simulink model "mars_rover_ex_1b"  (R2023a)
settings: Solver=ode23t  StartTime=0.0  StopTime=Rover.simStopTimeEx1b  FixedStep=1e-2  MaxStep=0.1  RelTol=1e-3  AbsTol=1e-3  EnableMultiTasking=on
StartFcn:
  | mars_rover_ex1b_sim_callback
model workspace (MATLAB code in the model file):
  | addpath("mars_rover_helpers");
  | % Load Rover Arm model for IK
  | mdlpath = ['mars_rover_data',filesep,'mars_rover_arm'];
  | load_system(mdlpath);
  | 
  | imdata = zeros(3,3,3);
  | 
  | % Temp
  | Kp_steer = 1;
  | Ki_steer = 1;
  | Kd_steer = 1;
  | 
  | Kp = 1;
  | Ki = 1;
  | Kd = 1;
values from neighbouring files (symbols this model uses):
  cam_base_angle = 0    [mars_rover_params.m]
  cam_target_angle = 20    [mars_rover_params.m]
  mapData = false(197,200)    [mars_rover_params.m]    (also in mars_rover_startup.m)
  roverPath = app.rover_path    [NavigateOnMars.m]    (also in mars_rover_params.m = rover_path1)
undefined symbols (not defined in the file or in its folder): Arm, armJointAng, armJointTrqs, cameraData, eeConfig, pose, Rover, rover_path_ex1, sampleLocation, steerAng, steerTrqs, Terrain, vSpeed, Wheel1_G, Wheel2_G, Wheel3_G, Wheel4_G, Wheel5_G, Wheel6_G, wheelTrqs, wSpeeds, X, Y, Z
libraries: sm_lib x238, nesl_utility x80, slpidlib x3, simulink x3, simulink_extras x2, robotcorelib x1, robotalgslib x1
(part 9 of 9)

== system mars_rover_ex_1b/Mars Rover Plant/Rover Plant Model/Rover /Wheels/SteeringBracketLF ==
  File Solid5 : sm_lib/Body Elements/File Solid  ExtGeomFileName=mobility_steering_bracket.stl  UnitType=Custom  ExtGeomFileUnits=cm  StepReaderType=HEX  ExportConvexHullGeometry=off  InertiaType=CalculateFromGeometry  Mass=0  MassUnits=kg  CenterOfMass=[0 0 0]  CenterOfMassUnits=m  MomentsOfInertia=[1 1 1]*0  MomentsOfInertiaUnits=kg*m^2  ProductsOfInertia=[0 0 0]  ProductsOfInertiaUnits=kg*m^2  BasedOnType=Density  Density=1000  DensityUnits=kg/m^3  DoExposeReferenceFrame=on  SerializedFrames=<Frames/>  GraphicType=FromGeometry  MarkerShape=Sphere  MarkerSize=10  GraphicVisPropType=AdvancedVisualProperties  GraphicDiffuseColor=[0.2 0.2 0.2]  GraphicSpecularColor=[1 1 1 1.0]  GraphicAmbientColor=[0.15 0.15 0.15 1.0]  GraphicEmissiveColor=[0.0 0.0 0.0 1.0]  GraphicShininess=90  GraphicOpacity=1.0
  Reference Frame : sm_lib/Frames and Transforms/Reference Frame
  Rigid Transform : sm_lib/Frames and Transforms/Rigid Transform  TranslationMethod=Cartesian  TranslationStandardOffset=0  TranslationStandardOffsetUnits=m  TranslationStandardAxis=+Z  TranslationCartesianOffset=Rover.SB.SRJ_T  TranslationCartesianOffsetUnits=m  TranslationROffset=0  TranslationROffsetUnits=m  TranslationZOffset=0  TranslationZOffsetUnits=m  TranslationThetaOffset=0  TranslationThetaOffsetUnits=deg  RotationMethod=RotationMatrix  RotationAngleUnits=deg  RotationStandardAxis=+Z  RotationAngle=0.0  RotationArbitraryAxis=[0 0 1]  FollAlignAxisA=+X  BaseAlignAxisA=+Y  FollAlignAxisB=+Y  BaseAlignAxisB=+Z  RotationSequenceAxes=FollowerAxes  RotationSequence=XYX  RotationSequenceAngles=[0 0 0]  RotationSequenceAnglesUnits=deg  RotationMatrix=Rover.SB.SRJ_R  Quaternion=[1 0 0 0]
  Rigid Transform1 : sm_lib/Frames and Transforms/Rigid Transform  TranslationMethod=Cartesian  TranslationStandardOffset=0  TranslationStandardOffsetUnits=m  TranslationStandardAxis=+Z  TranslationCartesianOffset=Rover.SB.WRJ_T  TranslationCartesianOffsetUnits=m  TranslationROffset=0  TranslationROffsetUnits=m  TranslationZOffset=0  TranslationZOffsetUnits=m  TranslationThetaOffset=0  TranslationThetaOffsetUnits=deg  RotationMethod=RotationMatrix  RotationAngleUnits=deg  RotationStandardAxis=+Z  RotationAngle=0.0  RotationArbitraryAxis=[0 0 1]  FollAlignAxisA=+X  BaseAlignAxisA=+Y  FollAlignAxisB=+Y  BaseAlignAxisB=+Z  RotationSequenceAxes=FollowerAxes  RotationSequence=XYX  RotationSequenceAngles=[0 0 0]  RotationSequenceAnglesUnits=deg  RotationMatrix=Rover.SB.WRJ_R  Quaternion=[1 0 0 0]
  SRJ : PMIOPort  Side=Left
  WRJ : PMIOPort  Port=2  Side=Right
  connections:
  Rigid Transform/RConn1 -- SRJ/RConn1
  WRJ/RConn1 -- Rigid Transform1/RConn1
  File Solid5/RConn1 -- Reference Frame/RConn1 -- Rigid Transform1/LConn1 -- Rigid Transform/LConn1

== system mars_rover_ex_1b/Mars Rover Plant/Rover Plant Model/Rover /Wheels/SteeringBracketRB ==
  File Solid5 : sm_lib/Body Elements/File Solid  ExtGeomFileName=mobility_steering_bracket.stl  UnitType=Custom  ExtGeomFileUnits=cm  StepReaderType=HEX  ExportConvexHullGeometry=off  InertiaType=CalculateFromGeometry  Mass=0  MassUnits=kg  CenterOfMass=[0 0 0]  CenterOfMassUnits=m  MomentsOfInertia=[1 1 1]*0  MomentsOfInertiaUnits=kg*m^2  ProductsOfInertia=[0 0 0]  ProductsOfInertiaUnits=kg*m^2  BasedOnType=Density  Density=1000  DensityUnits=kg/m^3  DoExposeReferenceFrame=on  SerializedFrames=<Frames/>  GraphicType=FromGeometry  MarkerShape=Sphere  MarkerSize=10  GraphicVisPropType=AdvancedVisualProperties  GraphicDiffuseColor=[0.2 0.2 0.2]  GraphicSpecularColor=[1 1 1 1.0]  GraphicAmbientColor=[0.15 0.15 0.15 1.0]  GraphicEmissiveColor=[0.0 0.0 0.0 1.0]  GraphicShininess=90  GraphicOpacity=1.0
  Reference Frame : sm_lib/Frames and Transforms/Reference Frame
  Rigid Transform : sm_lib/Frames and Transforms/Rigid Transform  TranslationMethod=Cartesian  TranslationStandardOffset=0  TranslationStandardOffsetUnits=m  TranslationStandardAxis=+Z  TranslationCartesianOffset=Rover.SB.SRJ_T  TranslationCartesianOffsetUnits=m  TranslationROffset=0  TranslationROffsetUnits=m  TranslationZOffset=0  TranslationZOffsetUnits=m  TranslationThetaOffset=0  TranslationThetaOffsetUnits=deg  RotationMethod=RotationMatrix  RotationAngleUnits=deg  RotationStandardAxis=+Z  RotationAngle=0.0  RotationArbitraryAxis=[0 0 1]  FollAlignAxisA=+X  BaseAlignAxisA=+Y  FollAlignAxisB=+Y  BaseAlignAxisB=+Z  RotationSequenceAxes=FollowerAxes  RotationSequence=XYX  RotationSequenceAngles=[0 0 0]  RotationSequenceAnglesUnits=deg  RotationMatrix=Rover.SB.SRJ_R  Quaternion=[1 0 0 0]
  Rigid Transform1 : sm_lib/Frames and Transforms/Rigid Transform  TranslationMethod=Cartesian  TranslationStandardOffset=0  TranslationStandardOffsetUnits=m  TranslationStandardAxis=+Z  TranslationCartesianOffset=Rover.SB.WRJ_T  TranslationCartesianOffsetUnits=m  TranslationROffset=0  TranslationROffsetUnits=m  TranslationZOffset=0  TranslationZOffsetUnits=m  TranslationThetaOffset=0  TranslationThetaOffsetUnits=deg  RotationMethod=RotationMatrix  RotationAngleUnits=deg  RotationStandardAxis=+Z  RotationAngle=0.0  RotationArbitraryAxis=[0 0 1]  FollAlignAxisA=+X  BaseAlignAxisA=+Y  FollAlignAxisB=+Y  BaseAlignAxisB=+Z  RotationSequenceAxes=FollowerAxes  RotationSequence=XYX  RotationSequenceAngles=[0 0 0]  RotationSequenceAnglesUnits=deg  RotationMatrix=Rover.SB.WRJ_R  Quaternion=[1 0 0 0]
  SRJ : PMIOPort  Side=Left
  WRJ : PMIOPort  Port=2  Side=Right
  connections:
  Rigid Transform/LConn1 -- Rigid Transform1/LConn1 -- Reference Frame/RConn1 -- File Solid5/RConn1
  WRJ/RConn1 -- Rigid Transform1/RConn1
  Rigid Transform/RConn1 -- SRJ/RConn1

== system mars_rover_ex_1b/Mars Rover Plant/Rover Plant Model/Rover /Wheels/SteeringBracketRF ==
  File Solid5 : sm_lib/Body Elements/File Solid  ExtGeomFileName=mobility_steering_bracket.stl  UnitType=Custom  ExtGeomFileUnits=cm  StepReaderType=HEX  ExportConvexHullGeometry=off  InertiaType=CalculateFromGeometry  Mass=0  MassUnits=kg  CenterOfMass=[0 0 0]  CenterOfMassUnits=m  MomentsOfInertia=[1 1 1]*0  MomentsOfInertiaUnits=kg*m^2  ProductsOfInertia=[0 0 0]  ProductsOfInertiaUnits=kg*m^2  BasedOnType=Density  Density=1000  DensityUnits=kg/m^3  DoExposeReferenceFrame=on  SerializedFrames=<Frames/>  GraphicType=FromGeometry  MarkerShape=Sphere  MarkerSize=10  GraphicVisPropType=AdvancedVisualProperties  GraphicDiffuseColor=[0.2 0.2 0.2]  GraphicSpecularColor=[1 1 1 1.0]  GraphicAmbientColor=[0.15 0.15 0.15 1.0]  GraphicEmissiveColor=[0.0 0.0 0.0 1.0]  GraphicShininess=90  GraphicOpacity=1.0
  Reference Frame : sm_lib/Frames and Transforms/Reference Frame
  Rigid Transform : sm_lib/Frames and Transforms/Rigid Transform  TranslationMethod=Cartesian  TranslationStandardOffset=0  TranslationStandardOffsetUnits=m  TranslationStandardAxis=+Z  TranslationCartesianOffset=Rover.SB.SRJ_T  TranslationCartesianOffsetUnits=m  TranslationROffset=0  TranslationROffsetUnits=m  TranslationZOffset=0  TranslationZOffsetUnits=m  TranslationThetaOffset=0  TranslationThetaOffsetUnits=deg  RotationMethod=RotationMatrix  RotationAngleUnits=deg  RotationStandardAxis=+Z  RotationAngle=0.0  RotationArbitraryAxis=[0 0 1]  FollAlignAxisA=+X  BaseAlignAxisA=+Y  FollAlignAxisB=+Y  BaseAlignAxisB=+Z  RotationSequenceAxes=FollowerAxes  RotationSequence=XYX  RotationSequenceAngles=[0 0 0]  RotationSequenceAnglesUnits=deg  RotationMatrix=Rover.SB.SRJ_R  Quaternion=[1 0 0 0]
  Rigid Transform1 : sm_lib/Frames and Transforms/Rigid Transform  TranslationMethod=Cartesian  TranslationStandardOffset=0  TranslationStandardOffsetUnits=m  TranslationStandardAxis=+Z  TranslationCartesianOffset=Rover.SB.WRJ_T  TranslationCartesianOffsetUnits=m  TranslationROffset=0  TranslationROffsetUnits=m  TranslationZOffset=0  TranslationZOffsetUnits=m  TranslationThetaOffset=0  TranslationThetaOffsetUnits=deg  RotationMethod=RotationMatrix  RotationAngleUnits=deg  RotationStandardAxis=+Z  RotationAngle=0.0  RotationArbitraryAxis=[0 0 1]  FollAlignAxisA=+X  BaseAlignAxisA=+Y  FollAlignAxisB=+Y  BaseAlignAxisB=+Z  RotationSequenceAxes=FollowerAxes  RotationSequence=XYX  RotationSequenceAngles=[0 0 0]  RotationSequenceAnglesUnits=deg  RotationMatrix=Rover.SB.WRJ_R  Quaternion=[1 0 0 0]
  SRJ : PMIOPort  Side=Left
  WRJ : PMIOPort  Port=2  Side=Right
  connections:
  Rigid Transform/RConn1 -- SRJ/RConn1
  WRJ/RConn1 -- Rigid Transform1/RConn1
  File Solid5/RConn1 -- Reference Frame/RConn1 -- Rigid Transform1/LConn1 -- Rigid Transform/LConn1

== system mars_rover_ex_1b/Mars Rover Plant/Rover Plant Model/Rover Pose Sensing/Kalman Filter/accelerometer ==
  Constant3 : Constant  Value=[0 0 3.72076]
  Ideal Sensor : sm_lib/Frames and Transforms/Transform Sensor  MeasurementFrame=NonRotatingFollower  RotationSequence=XYX  SenseAngle=off  SenseAxis=off  SenseQ=off  SenseR=on  SenseRotationSequence=off  SenseOmegaX=off  SenseOmegaY=off  SenseOmegaZ=off  SenseQDot=off  SenseRDot=off  SenseRotationSequenceDot=off  SenseAlphaX=off  SenseAlphaY=off  SenseAlphaZ=off  SenseQDDot=off  SenseRDDot=off  SenseX=off  SenseY=off  SenseZ=off  SenseRad=off  SenseAzim=off  SenseDist=off  SenseInc=off  SenseXDot=off  SenseYDot=off  SenseZDot=off  SenseRadDot=off  SenseAzimDot=off  SenseDistDot=off  SenseIncDot=off  SenseXDDot=on  SenseYDDot=on  SenseZDDot=on  SenseRadDDot=off  SenseAzimDDot=off  SenseDistDDot=off  SenseIncDDot=off
  Matrix Multiply : Product  Multiplication=Matrix(*)
  Mux : Mux  Inputs=3
  PS-Simulink Converter{6,8..10} (4 alike) : nesl_utility/PS-Simulink Converter  PhysicalDomain=network_engine_domain  SubClassName=ps_output  LeftPortType=input  RightPortType=output  PseudoPeriodic=off  Frequencies=[]  VectorFormat=inherit  Unit=inherit  AffineConversion=off
  Sensor Noise : RandomNumber  Variance=0.01  SampleTime=1
  Sum : Sum  Inputs=++|
  Sum1 : Sum  Inputs=++|
  Transpose : Math  Operator=transpose
  Rover : PMIOPort  Side=Right
  World : PMIOPort  Port=2  Side=Left
  Accelerometer Readings : Outport
  Direction Cosine Matrix : Outport  Port=2
  wires:
  PS-Simulink Converter9/1 -> Mux/3
  Mux/1 -> Sum/2
  Matrix Multiply/1 -> Sum/1
  PS-Simulink Converter6/1 -> Mux/1
  PS-Simulink Converter10/1 -> Direction Cosine Matrix/1, Transpose/1
  PS-Simulink Converter8/1 -> Mux/2
  Transpose/1 -> Matrix Multiply/1
  Constant3/1 -> Matrix Multiply/2
  Sensor Noise/1 -> Sum1/1
  Sum/1 -> Sum1/2
  Sum1/1 -> Accelerometer Readings/1
  connections:
  PS-Simulink Converter10/LConn1 -- Ideal Sensor/RConn2
  PS-Simulink Converter8/LConn1 -- Ideal Sensor/RConn4
  PS-Simulink Converter9/LConn1 -- Ideal Sensor/RConn5
  Ideal Sensor/RConn1 -- Rover/RConn1
  PS-Simulink Converter6/LConn1 -- Ideal Sensor/RConn3
  Ideal Sensor/LConn1 -- World/RConn1

== system mars_rover_ex_1b/Control/Rover Control/Rover Path Planning And Control/hold/RoverStopTime/Enabled Subsystem1 ==
  In1 : Inport
  Enable : EnablePort
  Out1 : Outport
  wires:
  In1/1 -> Out1/1

== matlab function mars_rover_ex_1b/Mars Rover Plant/Rover Plant Model/Rover Pose Sensing/Kalman Filter/Pose Estimation Outputs ==
  settings: updateMethod=DISCRETE  sampleTime=10
  data: plannedPath input; plannedPath_out output; estimatedXYStates input; estimatedXYStates_out output
function [plannedPath_out, estimatedXYStates_out]= fcn(plannedPath,estimatedXYStates)

plannedPath_out = plannedPath;
estimatedXYStates_out = estimatedXYStates;
end

== matlab function mars_rover_ex_1b/Control/Rover Control/Rover Path Planning And Control/Trapezoidal Vel Profile ==
  data: linVel input; t input; t1 input; lin_Vel_out output; accel input; deaccelStartTime input
function lin_Vel_out = fcn(linVel,t,t1,accel,deaccelStartTime)
% Function to create a trapezoidal profile for rover's desired linear
% velocity

t2 = linVel/accel + t1;
t3 = deaccelStartTime + 0.2;
tf = linVel/accel + t3;

if t>=t1 && t<t2 
    lin_Vel_out = accel*(t-t1);

elseif t>=t2 && t < t3 
    lin_Vel_out = linVel;

elseif t>= t3 && t < tf 
    lin_Vel_out = linVel-accel*(t-t3);

else
    lin_Vel_out = 0;    
end


end

== matlab function mars_rover_ex_1b/Control/Rover Control/Rover Path Planning And Control/Ackerman Steer Angle/Ackerman Steering Angle Formulation ==
  data: delta input; LFsteerAng output; L input; RFsteerAng output; d input; R output; L_R output; R_R output
function [LFsteerAng,RFsteerAng,R,L_R,R_R] = fcn(delta,L,d)
% Function to compute ackerman steering angles from a bicycle steer angle.

R = L/tand(abs(delta));

if delta < 0
    LFsteerAng = atan2d(L,(R+d/2));
    RFsteerAng = atan2d(L,(R-d/2));
    L_R = (R+d/2);
    R_R = (R-d/2);
else
    LFsteerAng = -atan2d(L,(R-d/2));
    RFsteerAng = -atan2d(L,(R+d/2));
    L_R = (R-d/2);
    R_R = (R+d/2);
end

end

== matlab function mars_rover_ex_1b/Control/Rover Control/Rover Path Planning And Control/Chassis Velocity To Wheel Speed ==
  data: desChassisSpeed input; wheel_speed_LF output; wheel_r input; steer_ang input; wheel_speed_LM output; wheel_speed_LB output; R input; L input; L_R input; R_R input; wheel_speed_RF output; wheel_speed_RM output; wheel_speed_RB output
function [wheel_speed_LF,wheel_speed_LM,wheel_speed_LB,...
    wheel_speed_RF,wheel_speed_RM,wheel_speed_RB] = fcn(desChassisSpeed,wheel_r,steer_ang,R,L,L_R,R_R)
% Function to compute wheel speed from a desired linear velocity and
% desired path.

if any(abs(steer_ang) > 0)

    wheel_speed_LF = (desChassisSpeed/wheel_r)*sqrt(L_R^2 + L^2)/R;
    wheel_speed_LM = desChassisSpeed * L_R/(R*wheel_r);
    wheel_speed_LB = (desChassisSpeed/wheel_r)*sqrt(L_R^2 + L^2)/R;
    wheel_speed_RF = -(desChassisSpeed/wheel_r)*sqrt(R_R^2 + L^2)/R;
    wheel_speed_RM = -desChassisSpeed * R_R/(R*wheel_r);
    wheel_speed_RB = -(desChassisSpeed/wheel_r)*sqrt(R_R^2 + L^2)/R;

else
    wheel_speed_LF = desChassisSpeed / wheel_r;
    wheel_speed_LM = desChassisSpeed / wheel_r;
    wheel_speed_LB = desChassisSpeed / wheel_r;
    wheel_speed_RF = -desChassisSpeed / wheel_r;
    wheel_speed_RM = -desChassisSpeed / wheel_r;
    wheel_speed_RB = -desChassisSpeed / wheel_r;
end

end

== matlab function mars_rover_ex_1b/Control/Manipulator Control/ Trajectory Planner/Planner Subsystem/Task Scheduler ==
  settings: updateMethod=DISCRETE
  data: wayPts output; reset_t output; samplePickCmd output; sampleDropCmd output; actJointAngles input; desJointAngles input; samplePickSense input; sampleDropSense input; currentTime input; stop output
function [wayPts,reset_t,samplePickCmd,sampleDropCmd,stop]  = fcn(actJointAngles,desJointAngles,samplePickSense,sampleDropSense,currentTime)
% This function plans the top level tasks for the arm. The end effector goal
% and sample interaction joint configuration modes depend on the current task mode.
%
% mode 0: home/initial position (waypt 1) (samplePickCmd Off)
% mode 1-2: move to the position close the sample (waypt 3 via waypt 2) (samplePickCmd Off)
% mode 3-4 : move to sample position and pick up sample (waypt 4) (samplePickCmd On)
% mode 5 : move back to the position close the sample (waypt 3) (samplePickCmd On)
% mode 6 : move to the position close to the sample storage unit (waypt 5) (samplePickCmd On)
% mode 7-8 : move to sample storage position and drop/collect sample (waypt 6) (sampleDropCmd On)
% mode 9 : move back to the position close to the sample storage unit (samplePickCmd,sampleDropCmd On)
% mode 10-11 :move to home position 

maxErrPos = 0.5;
actJointAngles =actJointAngles';
persistent mode resetTime
stop = 0;
if isempty(mode)
    mode = 0;
    resetTime = 0;
end

reset_t =  resetTime;

switch mode

    case 0
        % Home Position
        wayPts = [desJointAngles(1,:);desJointAngles(1,:)];
        samplePickCmd = false;
        sampleDropCmd = false;

        if all(abs(actJointAngles-desJointAngles(1,:)) < maxErrPos)
            resetTime = currentTime;
            if sampleDropSense == 1
                mode = 0;
            else
                mode = 1;
            end
        end

    case 1
        
        wayPts = desJointAngles(1:2,:);
        samplePickCmd = false;
        sampleDropCmd = false;

        if all(abs(actJointAngles-desJointAngles(2,:)) < maxErrPos)
            resetTime = currentTime;
            mode = 2;
        end

    case 2
        % Move to the position close the sample
        wayPts = desJointAngles(2:3,:);
        samplePickCmd = false;
        sampleDropCmd = false;

        if all(abs(actJointAngles-desJointAngles(3,:)) < maxErrPos)
            resetTime = currentTime;
            mode = 3;
        end

    case 3
        % Move to sample position
        wayPts = desJointAngles(3:4,:);
        samplePickCmd = false;
        sampleDropCmd = false;

        if all(abs(actJointAngles-desJointAngles(4,:)) < maxErrPos)
            resetTime = currentTime;
            mode = 4;
        end

    case 4
        % Stay at sample position and pick up the sample
        wayPts = [desJointAngles(4,:); desJointAngles(4,:)];
        samplePickCmd = true;
        sampleDropCmd = false;

        if all(abs(actJointAngles-desJointAngles(4,:)) < maxErrPos) && samplePickSense == 1
            resetTime = currentTime;
            mode = 5;
        end

    case 5
        % Move back to the position close to the sample
        wayPts = desJointAngles(4:-1:3,:);
        samplePickCmd = true;
        sampleDropCmd = false;

        if all(abs(actJointAngles-desJointAngles(3,:)) < maxErrPos)
            resetTime = currentTime;
            mode = 6;
        end


    case 6
        % Move the position close to the sample storage unit
        wayPts = [desJointAngles(3,:) ;desJointAngles(5,:)];
        samplePickCmd = true;
        sampleDropCmd = false;

        if all(abs(actJointAngles-desJointAngles(5,:)) < maxErrPos)
            resetTime = currentTime;
            mode = 7;
        end

    case 7
        % Move to the sample storage unit position
        wayPts = desJointAngles(5:6,:);
        sampleDropCmd = false;
        samplePickCmd = true;

        if all(abs(actJointAngles-desJointAngles(6,:)) < maxErrPos)
            resetTime = currentTime;
            mode = 8;
        end

    case 8
        % Stay at sample drop position, drop and collect the sample
        wayPts = [desJointAngles(6,:);desJointAngles(6,:)];

        sampleDropCmd = true;
        samplePickCmd = true;

        if (all(abs(actJointAngles-desJointAngles(6,:)) < maxErrPos)) && sampleDropSense == 1
            resetTime = currentTime;
            mode = 9;
        end

    case 9
        % Move back to the position close to the sample storage unit
        wayPts = desJointAngles(6:-1:5,:);
        sampleDropCmd = true;
        samplePickCmd = true;

        if all(abs(actJointAngles-desJointAngles(5,:)) < maxErrPos)
            resetTime = currentTime;
            mode = 10;
        end

    case 10
        % Move to home position via waypt 2
        wayPts = [desJointAngles(5,:); desJointAngles(7,:)];
        sampleDropCmd = true;
        samplePickCmd = true;

        if all(abs(actJointAngles-desJointAngles(7,:)) < maxErrPos)
            resetTime = currentTime;
            mode = 11;
        end

    case 11
        % Move to home position
        wayPts = [desJointAngles(7,:); desJointAngles(1,:)];
        sampleDropCmd = true;
        samplePickCmd = true;

        if all(abs(actJointAngles-desJointAngles(1,:)) < maxErrPos)
            resetTime = currentTime;           
            mode = 12;
        end
   
    case 12
        % Mission Complete
        wayPts = [desJointAngles(7,:); desJointAngles(1,:)];
        sampleDropCmd = true;
        samplePickCmd = true;
        mode = 12;
        stop = 1;
    otherwise
        error('invalid mode');

end

end

== matlab function mars_rover_ex_1b/Control/Manipulator Control/ Trajectory Planner/Planner Subsystem/Inverse Kinematics ==
  data: jointSpaceWayPts output; eePoseDes input; eeIgs input; samplePosition input; prevWayPts input
function  jointSpaceWayPts = fcn(eePoseDes,eeIgs,samplePosition,prevWayPts)
% Wrapper around sm_mars_rover_arm_ik.m
% Takes end effector targets and initial guesses and returns all the
% actuator positions corresponding to each target.

coder.extrinsic("mars_rover_arm_ik");

jointSpaceWayPts = zeros(7,6); %#ok<PREALL> 

% End effector Targets and initial guesses derived from sample location
samplePose = [samplePosition 175 0 91];
sample_position_eef = samplePose;
sample_position_eef_ig = [90.0000 -200.0000   90.0000   40.0000  170.0000  -10.0000];%[90   -200  160  90 170 -60];
sample_pos_init_eef = [sample_position_eef(1) sample_position_eef(2) sample_position_eef(3)+0.1 sample_position_eef(4) sample_position_eef(5) sample_position_eef(6)];
sample_pos_init_eef_ig = [90.0000 -200.0000   90.0000   40.0000  170.0000  -10.0000];%[90   -200  160  90 170 0];

% Combine precomputed end effector targets (waypts 1,2,5,6) with the
% ones derived from sample location (waypts 3,4) to create a set of
% task space waypoints for planning the trajectory.

EndEffTargets = ... 
    [eePoseDes(1,:);...% Waypt 1,(HomePos)
     eePoseDes(2,:);...% Waypt 2
    sample_pos_init_eef;...% Waypt 3,(Position near sample)
    sample_position_eef;...% Waypt 4 (Sample position)
    eePoseDes(3,:);... % Waypt 5,(Position near storage unit)
    eePoseDes(4,:);...% Waypt 6,(Sample storage position)
    eePoseDes(5,:);...
    ];

EndEffIgs = ...
     [eeIgs(1,:);...
     eeIgs(2,:);...
     sample_pos_init_eef_ig ;...  
     sample_position_eef_ig;...
     eeIgs(3,:);...
     eeIgs(4,:);...
     eeIgs(5,:);...
    ];

% Obtain joint space waypoints by calling IK for each end effector target
if prevWayPts == zeros(7,6)
[jointSpaceWayPts,solvedFlag] =  mars_rover_arm_ik(EndEffTargets,EndEffIgs); %#ok<ASGLU> 
else
jointSpaceWayPts = prevWayPts;
end

end

== matlab function mars_rover_ex_1b/Mars Rover Plant/Manipulator Plant Model/SampleGeneration/Subsystem/MATLAB Function ==
  data: roverPose input; sampleLoc output; terrainPts input
function sampleLoc = fcn(roverPose,terrainPts)
sampleLoc = zeros(3,1);
coder.extrinsic("scatteredInterpolant");

    P_rs = [2.25; 0; 0];
    R_wr = eul2rotm([0 0 roverPose(3)],'XYZ');
    P_wr = [roverPose(1) roverPose(2) 0];

    P_ws = P_wr' + R_wr*P_rs;

    F = scatteredInterpolant(terrainPts(:,1),terrainPts(:,2),terrainPts(:,3));
    sampleLoc = [P_ws(1);P_ws(2);F(P_ws(1),P_ws(2))];


end

== matlab function mars_rover_ex_1b/Mars Rover Plant/Rover Plant Model/Rover Pose Sensing/Kalman Filter/Discrete-Time Linear Kalman Filter ==
  settings: updateMethod=DISCRETE  sampleTime=1
  data: accelerometerData input; EstPose output; DCMMat input; rover_initialPosition input; t input; wheelSpeed input; wheel_radius input; EstLinVel output; EstLinAccel output; linVelocity input
function [EstPose, EstLinVel, EstLinAccel]  = fcn(accelerometerData, DCMMat,rover_initialPosition, t, wheelSpeed, wheel_radius,linVelocity)
% Discrete-Time Kalman Filter Block to estimate the position, linear
% velocity and linear acceleration of the rover using the IMU data and
% wheel speed. The system is defined as follows in continuous time: x_dot =
% [0 0 0 1 0 0 0 0 0; 0 0 0 0 1 0 0 0 0; 0 0 0 0 0 1 0 0 0;...
%          0 0 0 0 0 0 1 0 0; 0 0 0 0 0 0 0 1 0; 0 0 0 0 0 0 0 0 1;... 0 0
%          0 0 0 0 0 0 0; 0 0 0 0 0 0 0 0 0; 0 0 0 0 0 0 0 0 0]*x + G*w;
% where, x = [x;y;z;xdot;ydot;zdot;x_ddot;y_ddot;z_ddot] w is process noise
% with covariance qNoise. G = [0;0;0;1;1;1;1;1;1]
%
% The measurement model is given by yk = H*x; H = [0 0 0 0 0 0 0 0 0;...
%      0 0 0 0 0 0 0 0 0;... 0 0 0 0 0 0 0 0 0;... 0 0 0 1 0 0 0 0 0;... 0
%      0 0 0 1 0 0 0 0;... 0 0 0 0 0 1 0 0 0;... 0 0 0 0 0 0 1 0 0;... 0 0
%      0 0 0 0 0 1 0;... 0 0 0 0 0 0 0 0 1];
%
% The discrete-time state matrix is given by F = [1 0 0 Ts 0 0 Ts^2/2 0
% 0;...
%          0 1 0 0 Ts 0 0 Ts^2/2 0;... 0 0 1 0 0 Ts 0 0 Ts^2/2;... 0 0 0 1
%          0 0 Ts 0 0;... 0 0 0 0 1 0 0 Ts 0;... 0 0 0 0 0 1 0 0 Ts;... 0 0
%          0 0 0 0 1 0 0;... 0 0 0 0 0 0 0 1 0;... 0 0 0 0 0 0 0 0 1];
% where Ts is time step

eul = rotm2eul(DCMMat,'XYZ');

g = -3.72076; % acceleration due to gravity in m/s^2
rNoise = 1e-5; % Sensor noise variance
qNoise = 5e-5; % Process Noise variance
G = [0;0;0;0;0;0;1;1;1];
x_ini = rover_initialPosition(1,1);
y_ini = rover_initialPosition(2,1);
z_ini = rover_initialPosition(3,1);

% Initialize
persistent t_prev xhat P P_propagated xhat_propagated xhatEst

if isempty(t_prev)
    t_prev = 0;
end

if isempty(xhatEst)
    xhatEst = [x_ini;y_ini;z_ini;zeros(6,1)];
end

if isempty(xhat_propagated)
    xhat_propagated = [x_ini;y_ini;z_ini;zeros(6,1)];
end

if isempty(xhat)
    xhat = [x_ini;y_ini;z_ini;zeros(6,1)];
end

if isempty(P_propagated)
    P_propagated = [0 0 0 0 0 0 0 0 0;...
        0 0 0 0 0 0 0 0 0;...
        0 0 0 0 0 0 0 0 0;...
        0 0 0 10 0 0 0 0 0;...
        0 0 0 0 10 0 0 0 0;...
        0 0 0 0 0 0 0 0 0;...
        0 0 0 0 0 0 1 0 0;...
        0 0 0 0 0 0 0 1 0;...
        0 0 0 0 0 0 0 0 0];
end

if isempty(P)
    P = [0 0 0 0 0 0 0 0 0;...
        0 0 0 0 0 0 0 0 0;...
        0 0 0 0 0 0 0 0 0;...
        0 0 0 10 0 0 0 0 0;...
        0 0 0 0 10 0 0 0 0;...
        0 0 0 0 0 0 0 0 0;...
        0 0 0 0 0 0 1 0 0;...
        0 0 0 0 0 0 0 1 0;...
        0 0 0 0 0 0 0 0 0];
end

Ts = t - t_prev; % Calculate time step

% Propagate States and Covariance Matrix Accelerometer Readings
accelerometerData_inertialFrame = DCMMat*[accelerometerData(1,1);accelerometerData(2,1);accelerometerData(3,1)] + [0;0;g];
ax = accelerometerData_inertialFrame(1,1);
ay = accelerometerData_inertialFrame(2,1);
az = accelerometerData_inertialFrame(3,1);

% Wheel odometry measurements assuming plannar assumption
omegaLM = wheelSpeed(2,1);
omegaRM = wheelSpeed(5,1);
% linVel_body = (wheel_radius*(abs(omegaLM) + abs(omegaRM))/2)*0.88;
% linVel = DCMMat*[linVel_body;0;0]; % linearVelocityXY
linVel = [linVelocity; 0];

F = [1 0 0 Ts 0 0 Ts^2/2 0 0;...
    0 1 0 0 Ts 0 0 Ts^2/2 0;...
    0 0 1 0 0 Ts 0 0 Ts^2/2;...
    0 0 0 1 0 0 Ts 0 0;...
    0 0 0 0 1 0 0 Ts 0;...
    0 0 0 0 0 1 0 0 Ts;...
    0 0 0 0 0 0 1 0 0;...
    0 0 0 0 0 0 0 1 0;...
    0 0 0 0 0 0 0 0 1]; % Transition Matrix

H = [0 0 0 0 0 0 0 0 0;...
    0 0 0 0 0 0 0 0 0;...
    0 0 0 0 0 0 0 0 0;...
    0 0 0 1 0 0 0 0 0;...
    0 0 0 0 1 0 0 0 0;...
    0 0 0 0 0 0 0 0 0;...
    0 0 0 0 0 0 1 0 0;...
    0 0 0 0 0 0 0 1 0;...
    0 0 0 0 0 0 0 0 0];

xhat_propagated = F*xhatEst; % propagated states

P_propagated = F*P*F' + G*qNoise*G'; % propagated covariance matrix

% Calculate Gain, K
R = [rNoise*1e-5 0 0 0 0 0 0 0 0;...
    0 rNoise*1e-5 0 0 0 0 0 0 0;...
    0 0 rNoise*1e-5 0 0 0 0 0 0;...
    0 0 0 rNoise*1e-1 0 0 0 0 0;...
    0 0 0 0 rNoise*1e-1 0 0 0 0;...
    0 0 0 0 0 rNoise*1e-1 0 0 0;...
    0 0 0 0 0 0 rNoise 0 0;...
    0 0 0 0 0 0 0 rNoise 0;...
    0 0 0 0 0 0 0 0 rNoise]; % rNoise*eye(9);
K = P_propagated*H'*inv(H*P_propagated*H' + R);

% Residual
x = xhat_propagated(1,1);
y = xhat_propagated(2,1);
z = xhat_propagated(3,1);
x_dot = linVel(1,1);
y_dot = linVel(2,1);
z_dot = linVel(3,1); % xhat_propagated(6,1);
x_ddot = ax;
y_ddot = ay;
z_ddot = az;

y = H*[x;y;z;x_dot;y_dot;z_dot;x_ddot;y_ddot;z_ddot] - H*xhat_propagated; % Residual

% Measurement Update (Compute Estimate)
xhat = xhat_propagated;
xhatEst = xhat + K*y; % Measurement update to compute the estimates

xEst = xhatEst(1,1);
yEst = xhatEst(2,1);
zEst = xhatEst(3,1);

x_dotEst = xhatEst(4,1);
y_dotEst = xhatEst(5,1);
z_dotEst = xhatEst(6,1);

x_ddotEst = xhatEst(7,1);
y_ddotEst = xhatEst(8,1);
z_ddotEst = xhatEst(9,1);

EstPose = [xEst;yEst];
EstLinVel = [x_dotEst; y_dotEst];
EstLinAccel = [x_ddotEst; y_ddotEst; z_ddotEst];

P = (eye(9) - K*H)*P_propagated;
t_prev = t;

== matlab function mars_rover_ex_1b/Online Planner/Online Planner/pathPlanner ==
  settings: sampleTime=0.1
  data: mapData input; refpath output [..200]; startLocation input; endLocation input; obstacleLocation input; initRoverPath input; newMapData output; correctedObsLoc output
function [refpath, newMapData,correctedObsLoc] = planRoverHybridAStar(mapData,startLocation,endLocation,obstacleLocation,initRoverPath)
initSize = size(initRoverPath);
refpath = zeros(initSize);
newMapData = false(197,200);
correctedObsLoc = zeros(size(obstacleLocation));
coder.extrinsic('planRoverHybridAStarWrapper');
coder.extrinsic('find')
coder.extrinsic('any')

% nonzero_ids = find(any(obstacleLocation,2));

disp('called')
[refpath,~,newMapData,correctedObsLoc] = planRoverHybridAStarWrapper(mapData,startLocation,endLocation,obstacleLocation,initRoverPath);   

end

== matlab function mars_rover_ex_1b/Perception/Deep Learning Object Detector/MLFB ==
  settings: updateMethod=DISCRETE  sampleTime=15
  data: image input; bboxes output size=[500 4]; scores output size=[500 1]
function [bboxes, scores] = objectDetector(image)
isSim = coder.target('sfun');
simSupported = false;
useExtrinsic = isSim && ~simSupported;
[bboxes, scores] = deep.blocks.internal.objectDetector(image, 'rockDetectorDL.mat', true, {'Threshold', 0.565, 'SelectStrongest', false}, {}, 500, true, false, true);
end

== matlab function mars_rover_ex_1b/Perception/depthEstimation ==
  settings: updateMethod=DISCRETE  sampleTime=30
  data: I_left input; I_right input; im_out output; in_bboxes input; obstacleWorldXYZ output size=[500 4] [..20000]; rover_translation input; rover_orientation input; cam_base_angle input; cam_target_angle input; obstacleDistance output size=[1 100]
function [im_out,obstacleWorldXYZ,obstacleDistance] = fcn(I_left,I_right,in_bboxes,rover_translation,rover_orientation,cam_base_angle,cam_target_angle)

im_out = uint8(zeros(420,560,3));
obstacleWorldXYZ = zeros(100,3);
obstacleDistance = zeros(1,100);
coder.extrinsic("mars_rover_stereo_vision");

if ~isempty(in_bboxes)
[im_out, obstacleWorldXYZ, obstacleDistance] = mars_rover_stereo_vision(I_left,I_right,in_bboxes,rover_translation,rover_orientation,cam_base_angle,cam_target_angle);
end


end

== matlab function mars_rover_ex_1b/Perception/rocksOnPath ==
  settings: updateMethod=DISCRETE  sampleTime=30
  data: scores input; obstacleWorldXYZ input; obstacleDistance input; roverPath input; rocksOnPath output; rePlanFlag output; mapData input
function [rocksOnPath ,rePlanFlag]= fcn(scores,obstacleWorldXYZ,obstacleDistance,roverPath,mapData)

% Create a circle with radius of 0.8 m and center at obstacleLocation

rocksOnPath = zeros(100,3);
rocks_path = zeros(100,3);
rePlanFlag = 0;
% roverPath = [roverPath_x roverPath_y];
k = 1;
map = binaryOccupancyMap(mapData,'resolution',5);

if any(obstacleDistance(:))

    for i = 1:size(obstacleWorldXYZ,1)

        if obstacleDistance(i) <= 3.5 && (scores(i) >= 0.565)

            x_rock = obstacleWorldXYZ(i,1);
            y_rock = obstacleWorldXYZ(i,2);
          
            for j = 1:size(roverPath,1)

                x_path = roverPath(j,1);
                y_path = roverPath(j,2);

                dist = sqrt((x_path-x_rock)^2 + (y_path-y_rock)^2);
                 if dist <= 1.4
                    rocks_path(k,:) = obstacleWorldXYZ(i,:);
                    rePlanFlag = 1;
                    k = k+1;
                end
              
            end
        end

    end
end

rocks_path = unique(rocks_path,'rows');

for r = 1:size(rocks_path,1)

    rocksOnPath(r,:) = rocks_path(r,:);

end


end

== matlab function mars_rover_ex_1b/Perception/sceneViewer/Left/LCam ==
  settings: updateMethod=DISCRETE  sampleTime=0.8
  data: rot_mat input; Camera_Z_ang output; Camera_pos output; Camera_rot output; Camera_target_ang output; x input; y input; z input; target_ang input
function [Camera_Z_ang, Camera_pos, Camera_rot, Camera_target_ang]= fcn(rot_mat,x,y,z,target_ang)

out = rotm2eul(rot_mat);
Camera_Z_ang = out(1);
Camera_pos = [x y z];
Camera_rot = rot_mat;
Camera_target_ang = target_ang;
end

== matlab function mars_rover_ex_1b/Perception/sceneViewer/Stereo_Left/drawScene/Camera ==
  settings: sampleTime=0.1
  data: Camera_Z_ang input; Camera_pos input; Camera_rot input; Camera_target_ang input; xg input; yg input; z_heights input; znew input; rover_path_x input; rover_path_y input; rover_path_z input; im output
 function im = fcn(Camera_Z_ang,...
                         Camera_pos,...
                         Camera_rot,...
                         Camera_target_ang,...
                         xg,yg,z_heights,znew,...
                         rover_path_x,rover_path_y,rover_path_z)
im = uint8(zeros(420,560,3));
coder.extrinsic('axes')
coder.extrinsic('figure')
coder.extrinsic('plotSurfaceForCamera')
coder.extrinsic('getframe')
coder.extrinsic('moveCamera');
coder.extrinsic('getfield');
coder.extrinsic('print');
coder.extrinsic('frame2im');
coder.extrinsic('imresize');
coder.extrinsic('imshow');

persistent  surface_ax  fig ; 

if isempty(surface_ax)
  
    % Plot the Surface plot in MATLAB.
    fh = findobj( 'Type', 'Figure', 'Name', 'LeftNavCam ');
    close(fh);
    fig = figure(21);
    set(fig,'Name','LeftNavCam');       
    set(fig, 'Visible', 'off');
    surface_ax = axes(fig,'XLim',[min(xg) max(xg)],'YLim',[min(yg) max(yg)],'ZLim',[0 8]);    
    plotSurfaceForCamera(surface_ax,xg,yg,z_heights,znew);
end

 moveCamera_L(surface_ax,Camera_Z_ang,Camera_pos,Camera_rot,Camera_target_ang);
 pause(0.005);
 frame = getframe(surface_ax);
 RGB = frame2im(frame);
 im = imresize(RGB,[420 560]);

end

== matlab function mars_rover_ex_1b/Perception/sceneViewer/Stereo_Left/theta_act ==
  data: u input; z output
function z  = fcn(u)
out = rotm2eul(u);
z = out(1);
% y = out(2);
%x = out(3);
end

== matlab function mars_rover_ex_1b/Perception/sceneViewer/Right/RCam ==
  settings: updateMethod=DISCRETE  sampleTime=0.8
  data: rot_mat input; Camera_Z_ang output; Camera_pos output; Camera_rot output; Camera_target_ang output; x input; y input; z input; target_ang input
function [Camera_Z_ang, Camera_pos, Camera_rot, Camera_target_ang]= fcn(rot_mat,x,y,z,target_ang)

out = rotm2eul(rot_mat);
Camera_Z_ang = out(1);
Camera_pos = [x y z];
Camera_rot = rot_mat;
Camera_target_ang = target_ang;
end

== matlab function mars_rover_ex_1b/Perception/sceneViewer/Stereo_Right/drawScene/Camera ==
  settings: sampleTime=0.1
  data: Camera_Z_ang input; Camera_pos input; Camera_rot input; Camera_target_ang input; xg input; yg input; z_heights input; znew input; rover_path_x input; rover_path_y input; rover_path_z input; im output
function im = fcn(Camera_Z_ang,...
    Camera_pos,...
    Camera_rot,...
    Camera_target_ang,...
    xg,yg,z_heights,znew,...
    rover_path_x,rover_path_y,rover_path_z)
im = uint8(zeros(420,560,3));
coder.extrinsic('axes')
coder.extrinsic('figure')
coder.extrinsic('plotSurfaceForCamera')
coder.extrinsic('getframe')
coder.extrinsic('moveCamera');
coder.extrinsic('getfield');
coder.extrinsic('print');
coder.extrinsic('frame2im');
coder.extrinsic('imresize');
coder.extrinsic('imshow');

persistent  surface_ax fig ;

if isempty(surface_ax)

    % Plot the Surface plot in MATLAB.
    fh = findobj( 'Type', 'Figure', 'Name', 'RightNavCam ');
    close(fh);
    fig = figure(22);%figure('Name','LeftNavCam');
    set(fig,'Name','RightNavCam');
    set(fig, 'Visible', 'off');
    surface_ax = axes(fig,'XLim',[min(xg) max(xg)],'YLim',[min(yg) max(yg)],'ZLim',[0 8]);
    plotSurfaceForCamera(surface_ax,xg,yg,z_heights,znew);
end

moveCamera_R(surface_ax,Camera_Z_ang,Camera_pos,Camera_rot,Camera_target_ang);
pause(0.005);
frame = getframe(surface_ax);
RGB = frame2im(frame);
im = imresize(RGB,[420 560]);

end

== matlab function mars_rover_ex_1b/Perception/sceneViewer/Stereo_Right/theta_act ==
  data: u input; z output
function z  = fcn(u)
out = rotm2eul(u);
z = out(1);
% y = out(2);
%x = out(3);
end

== matlab function mars_rover_ex_1b/Control/Rover Control/Rover Path Planning And Control/Target Dir To Bicycle Steer Angle/Rad2Deg ==
  data: u input; y output
function y = fcn(u)
y = rad2deg(u);

== matlab function mars_rover_ex_1b/Outputs/Rover Outputs/CalcSpeed ==
  data: u input; y output
function y = fcn(u)
y = sqrt(u(1)^2 + u(2)^2);
end

== matlab function mars_rover_ex_1b/Mars Rover Plant/Rover Plant Model/Rover Pose Sensing/Subsystem/theta_act ==
  data: u input; z output; y output; x output
function [z,y,x] = fcn(u)
out = quat2eul(u');
z = out(1);
y = out(2);
x = out(3);
end

== matlab function mars_rover_ex_1b/Mars Rover Plant/Rover Plant Model/Rover Pose Sensing/Subsystem/CalcSpeed ==
  data: u input; y output
function y = fcn(u)
y = sqrt(u(1)^2 + u(2)^2);
end

== matlab function mars_rover_ex_1b/Mars Rover Plant/Manipulator Plant Model/Rover Arm/rad2deg ==
  data: u input; y output
function y = fcn(u)

y = rad2deg(u);

== matlab function mars_rover_ex_1b/Control/Manipulator Control/ Trajectory Planner/SamplePickUpCmdLogic/DistanceError ==
  data: u input; flag output
function flag  = fcn(u)

distanceErr = sqrt(u(1)^2 + u(2)^2 +u(3)^2);

if distanceErr < 1e-2
    flag = true;
else
flag = false;
end

end

== matlab function mars_rover_ex_1b/Control/Manipulator Control/ Trajectory Planner/SampleDropOffCmdLogic/DistanceError ==
  data: u input; flag output
function flag  = fcn(u)

distanceErr = sqrt(u(1)^2 + u(2)^2 +u(3)^2);

if distanceErr < 1e-2
    flag = true;
else
flag = false;
end

end

== matlab function mars_rover_ex_1b/Mars Rover Plant/Rover Plant Model/Rover Pose Sensing/Kalman Filter/RoverNavTopView ==
  settings: updateMethod=DISCRETE  sampleTime=30
  data: pose input; pose_out output; originalPath input; originalPath_out output; xg input; yg input; z_heights input; znew input; xg_out output; yg_out output; z_heights_out output; znew_out output
function [pose_out,originalPath_out,xg_out,yg_out,z_heights_out,znew_out] = fcn(pose,originalPath,xg,yg,z_heights,znew)

pose_out = pose;
originalPath_out = originalPath;
xg_out = xg;
yg_out = yg;
z_heights_out = z_heights;
znew_out = znew;

end
